simulink model "MotorSpeedWithPID"  (R2021b)
settings: Solver=ode45  StartTime=0.0  StopTime=25  RelTol=1e-3
PreLoadFcn:
  | clear;
  | MS_PID
values from neighbouring files (symbols this model uses):
  MS_b_Cn = 0.1    [MS_PID.m]
  MS_J_Cn = 0.01    [MS_PID.m]
  MS_Ke_Cn = 0.01    [MS_PID.m]
  MS_Kt_Cn = 0.01    [MS_PID.m]
  MS_L_Cn = 0.5    [MS_PID.m]
  MS_R_Cn = 1    [MS_PID.m]
settings Model: Creator=sansh  LastModifiedBy=Dell-pc
settings SolverCC: AlgebraicLoopSolver=TrustRegion
settings DataIOCC: ReturnWorkspaceOutputs=off
settings DebuggingCC: SFMachineParentedDataDiag=warning  ArithmeticOperatorsInVariantConditions=warning
settings SFSimCC: SimUseLocalCustomCode=off  CustomCodeUndefinedFunction=UseInterfaceOnly
settings RTWCC: RTWUseLocalCustomCode=off
settings CodeAppCC: StateflowObjectComments=on

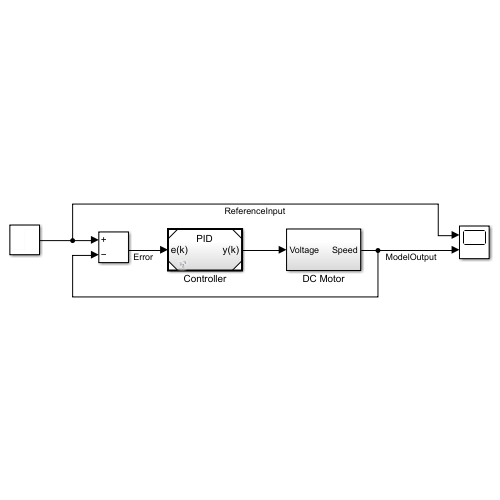
[thumbnail: Simulink's stored preview of the top-level diagram]
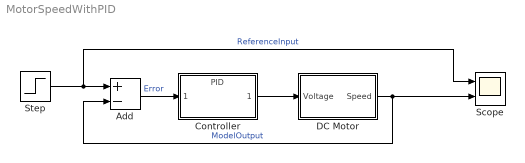
== system MotorSpeedWithPID ==
  Add : Sum  Inputs=+-
  Controller : ModelReference  ModelNameDialog=PID.slx  SimulationMode=Normal  ModelReferenceVersion=9.2
  DC Motor : Subsystem
  Scope : Scope  NumInputPorts=2
  Step : Step  SampleTime=0
  wires:
  Step/1 -> Scope/1, Add/1  "ReferenceInput"
  DC Motor/1(Speed) -> Add/2, Scope/2  "ModelOutput"
  Add/1 -> Controller/1  "Error"
  Controller/1 -> DC Motor/1(Voltage)

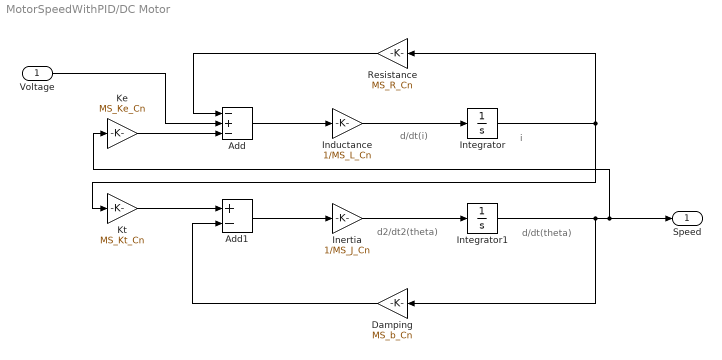
== system MotorSpeedWithPID/DC Motor ==
  note: i
  note: d/dt(i)
  note: d/dt(theta)
  note: d2/dt2(theta)
  Voltage : Inport
  Add : Sum  Inputs=-+-
  Add1 : Sum  Inputs=+-
  Damping : Gain  Gain=MS_b_Cn
  Inductance : Gain  Gain=1/MS_L_Cn
  Inertia : Gain  Gain=1/MS_J_Cn
  Integrator : Integrator
  Integrator1 : Integrator
  Ke : Gain  Gain=MS_Ke_Cn
  Kt : Gain  Gain=MS_Kt_Cn
  Resistance : Gain  Gain=MS_R_Cn
  Speed : Outport  VectorParamsAs1DForOutWhenUnconnected=off
  wires:
  Inductance/1 -> Integrator/1
  Integrator1/1 -> Damping/1, Speed/1, Ke/1
  Inertia/1 -> Integrator1/1
  Integrator/1 -> Resistance/1, Kt/1
  Kt/1 -> Add1/1
  Voltage/1 -> Add/2
  Resistance/1 -> Add/1
  Damping/1 -> Add1/2
  Ke/1 -> Add/3
  Add/1 -> Inductance/1
  Add1/1 -> Inertia/1
